simulink model "proyecto"  (R2017b)
settings: Solver=VariableStepAuto  StartTime=0.0  StopTime=3000  RelTol=1e-3
values from neighbouring files (symbols this model uses):
  A = [0 0 0 1 0 0 ... (first row only)    [Inicializar_proyecto.m]
  B = [0 0 ... (first row only)    [Inicializar_proyecto.m]
  C = [1 0 0 0 0 0 ... (first row only)    [Inicializar_proyecto.m]
  D = 2    [Deteccion.m]    (also in Inicializar_proyecto.m = [0 0)
  Elevacion = 50    [Inicializar_proyecto.m]    (also in simulacion_3d.m = 0)
  g = 9.81    [Inicializar_proyecto.m]
  Traslacion = 60    [Inicializar_proyecto.m]    (also in simulacion_3d.m = 0)
settings Model: Creator=Marco  LastModifiedBy=Marco

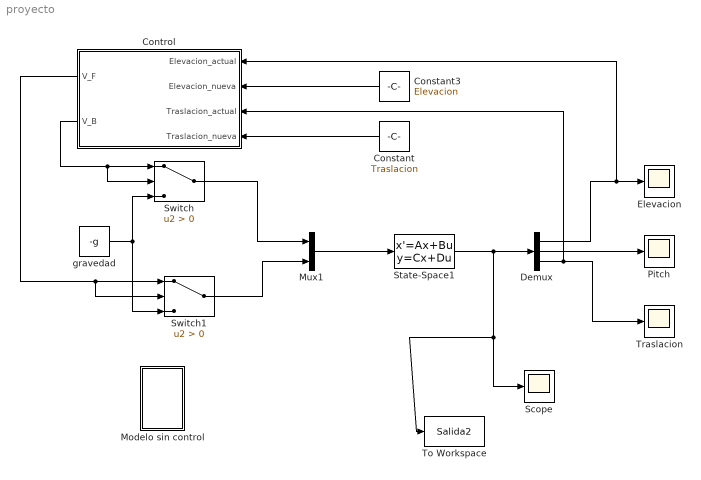
== system proyecto ==
  Constant : Constant  Value=Traslacion
  Constant3 : Constant  Value=Elevacion
  Control : MATLAB Function  TreatAsAtomicUnit=on
  Demux : Demux  Outputs=3
  Elevacion : Scope
  Modelo sin control : Subsystem
  Mux1 : Mux  Inputs=2
  Pitch : Scope
  Scope : Scope
  State-Space1 : StateSpace  A=A  B=B  C=C  D=D  InitialCondition=0
  Switch : Switch  Criteria=u2 > Threshold
  Switch1 : Switch  Criteria=u2 > Threshold
  To Workspace : ToWorkspace  VariableName=Salida2  SampleTime=-1
  Traslacion : Scope
  gravedad : Constant  Value=-g
  wires:
  gravedad/1 -> Switch1/3, Switch/3
  Mux1/1 -> State-Space1/1
  Switch1/1 -> Mux1/2
  Switch/1 -> Mux1/1
  Control/1(V_F) -> Switch1/2, Switch1/1
  Control/2(V_B) -> Switch/2, Switch/1
  Demux/1 -> Control/1(Elevacion_actual), Elevacion/1
  Demux/2 -> Pitch/1
  Constant3/1 -> Control/2(Elevacion_nueva)
  Constant/1 -> Control/4(Traslacion_nueva)
  Demux/3 -> Control/3(Traslacion_actual), Traslacion/1
  State-Space1/1 -> To Workspace/1, Scope/1, Demux/1

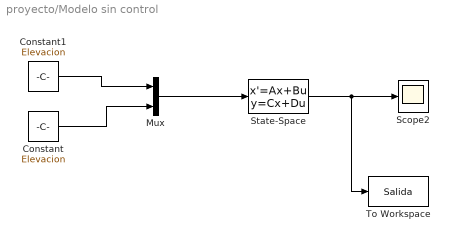
== system proyecto/Modelo sin control ==
  Constant : Constant  Value=Elevacion
  Constant1 : Constant  Value=Elevacion
  Mux : Mux  Inputs=2
  Scope2 : Scope
  State-Space : StateSpace  A=A  B=B  C=C  D=D  InitialCondition=0
  To Workspace : ToWorkspace  VariableName=Salida  SampleTime=-1
  wires:
  Mux/1 -> State-Space/1
  Constant/1 -> Mux/2
  Constant1/1 -> Mux/1
  State-Space/1 -> To Workspace/1, Scope2/1

== matlab function proyecto/Control ==
  data: Elevacion_actual input; V_F output; Elevacion_nueva input; V_B output; Traslacion_actual input; Traslacion_nueva input
function [V_F,V_B]= fcn(Elevacion_actual, Elevacion_nueva, Traslacion_actual, Traslacion_nueva)

V_nuevoB=0;
V_nuevoF=0;

delta_altura=Elevacion_actual-Elevacion_nueva;
delta_traslacion=Traslacion_actual-Traslacion_nueva;

if delta_altura<0
    V_nuevoB=10;
    V_nuevoF=10;
end
if delta_altura>0    
    V_nuevoB=-15;
    V_nuevoF=-15;
end

V_B=V_nuevoB;
V_F=V_nuevoF;

end
